simulink model "Lab2Part3"  (R2021b)
settings: Solver=VariableStepAuto  StartTime=0.0  StopTime=2  RelTol=1e-3
libraries: simulink x1
settings Model: Creator=gitan  LastModifiedBy=gitan

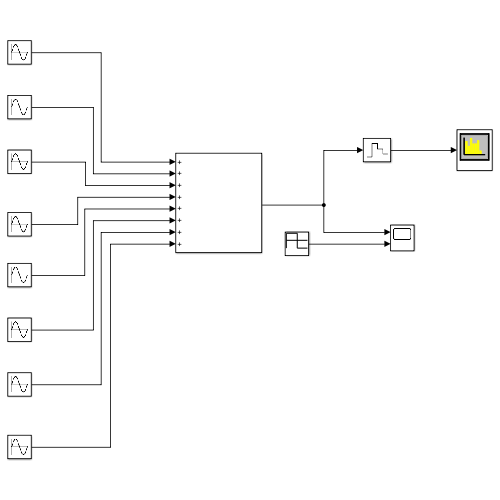
[thumbnail: Simulink's stored preview of the top-level diagram]
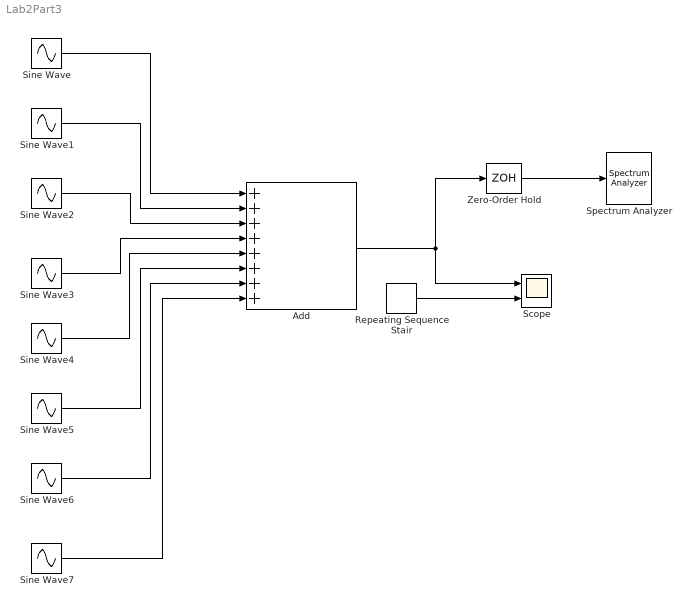
== system Lab2Part3 ==
  Add : Sum  Inputs=++++++++
  Repeating Sequence Stair : simulink/Sources/Repeating Sequence Stair  OutValues=[1 -1]  tsamp=1/64  OutMin=[]  OutMax=[]  OutDataTypeStr=double  OutputDataTypeScalingMode=double  OutDataType=fixdt(0,8)  ConRadixGroup=Best Precision: Vector-wise  OutScaling=2^-12
  Scope : Scope  NumInputPorts=2
  Sine Wave : Sin  Amplitude=4/3.14159  Frequency=32*2*3.14  SampleTime=0
  Sine Wave1 : Sin  Amplitude=4/(3*3.14)  Frequency=2*32*3.14*3  SampleTime=0
  Sine Wave2 : Sin  Amplitude=4/(5*3.14)  Frequency=2*32*3.14*5  SampleTime=0
  Sine Wave3 : Sin  Amplitude=4/(3.14*7)  Frequency=2*3.14*32*7  SampleTime=0
  Sine Wave4 : Sin  Amplitude=4/(9*3.14159)  Frequency=32*2*3.14 * 9  SampleTime=0
  Sine Wave5 : Sin  Amplitude=4/(11*3.14)  Frequency=2*32*3.14*11  SampleTime=0
  Sine Wave6 : Sin  Amplitude=4/(13*3.14)  Frequency=2*32*3.14*13  SampleTime=0
  Sine Wave7 : Sin  Amplitude=4/(3.14*15)  Frequency=2*3.14*32*15  SampleTime=0
  Spectrum Analyzer : SpectrumAnalyzer
  Zero-Order Hold : ZeroOrderHold  SampleTime=1/1024
  wires:
  Sine Wave/1 -> Add/1
  Sine Wave1/1 -> Add/2
  Sine Wave2/1 -> Add/3
  Sine Wave3/1 -> Add/4
  Add/1 -> Scope/1, Zero-Order Hold/1
  Zero-Order Hold/1 -> Spectrum Analyzer/1
  Repeating Sequence Stair/1 -> Scope/2
  Sine Wave4/1 -> Add/5
  Sine Wave5/1 -> Add/6
  Sine Wave6/1 -> Add/7
  Sine Wave7/1 -> Add/8
